simulink model "fuzzytest"  (R2016b)
settings: Solver=FixedStepAuto  StartTime=0.0  StopTime=100  FixedStep=Ts  RelTol=1e-3
values from neighbouring files (symbols this model uses):
  A_c = [0 1;0 0]    [fuzzysliding.m]    (also in fuzzytest.m)
  B_c = [0;Kx]    [fuzzysliding.m]    (also in fuzzytest.m = [0;K])
  C_c = [1 0]    [fuzzysliding.m]    (also in fuzzytest.m)
  D_c = 0    [fuzzysliding.m]    (also in fuzzytest.m)
  Ts = 0.02    [fuzzysliding.m]    (also in fuzzytest.m = 0.2)
libraries: simulink x1, fuzblock x1
settings Model: Creator=Ashraf  LastModifiedBy=Ashraf

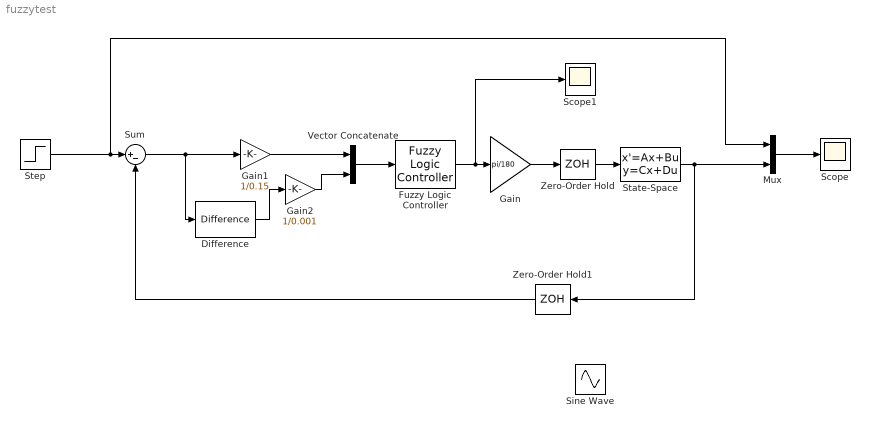
== system fuzzytest ==
  Difference : simulink/Discrete/Difference  ICPrevInput=0.0  OutMin=[]  OutMax=[]  OutDataType=fixdt(1, 16)  OutScaling=2^-10  DoSatur=off
  Fuzzy Logic Controller : fuzblock/Fuzzy Logic  Controller  fis='test3.fis'
  Gain : Gain  Gain=pi/180
  Gain1 : Gain  Gain=1/0.15
  Gain2 : Gain  Gain=1/0.001
  Mux : Mux  Inputs=2
  Scope : Scope
  Scope1 : Scope
  Sine Wave : Sin  SampleTime=0
  State-Space : StateSpace  A=A_c  B=B_c  C=C_c  D=D_c  X0=0
  Step : Step  Time=0  After=0.12  SampleTime=0
  Sum : Sum  Inputs=|+-
  Vector Concatenate : Concatenate
  Zero-Order Hold : ZeroOrderHold  SampleTime=Ts
  Zero-Order Hold1 : ZeroOrderHold  SampleTime=Ts
  wires:
  Zero-Order Hold/1 -> State-Space/1
  Gain/1 -> Zero-Order Hold/1
  Fuzzy Logic Controller/1 -> Scope1/1, Gain/1
  State-Space/1 -> Mux/2, Zero-Order Hold1/1
  Sum/1 -> Difference/1, Gain1/1
  Vector Concatenate/1 -> Fuzzy Logic Controller/1
  Zero-Order Hold1/1 -> Sum/2
  Gain1/1 -> Vector Concatenate/1
  Difference/1 -> Gain2/1
  Gain2/1 -> Vector Concatenate/2
  Mux/1 -> Scope/1
  Step/1 -> Mux/1, Sum/1
